simulink model "LQRC"  (R2020a)
settings: Solver=VariableStepAuto  StartTime=0  StopTime=30  FixedStep=0.01  MaxStep=0.1  MinStep=0.001  RelTol=1e-3  EnableMultiTasking=on
settings Model: Creator=s4khosra  LastModifiedBy=sashasen
settings DataIOCC: LimitDataPoints=on  SaveFormat=Array  ReturnWorkspaceOutputs=off
settings OptimizationCC: ExpressionDepthLimit=2147483647  LifeSpan=inf
settings DebuggingCC: AlgebraicLoopMsg=none  UnderspecifiedInitializationDetection=Classic  MergeDetectMultiDrivingBlocksExec=none  SolverPrmCheckMsg=warning  FcnCallInpInsideContextMsg=warning  AllowSymbolicDim=off  StateNameClashWarn=warning  SFUnexpectedBacktrackingDiag=warning  SFNoUnconditionalDefaultTransitionDiag=warning  SFExecutionAtInitializationDiag=none  ArithmeticOperatorsInVariantConditions=warning
settings HardwareCC: ProdBitPerPointer=32  ProdBitPerSizeT=32  ProdBitPerPtrDiffT=32  ProdLargestAtomicFloat=None  ProdIntDivRoundTo=Undefined  ProdEndianess=Unspecified  ProdWordSize=32  ProdHWDeviceType=32-bit Generic
settings ModelReferenceCC: PropagateSignalLabelsOutOfModel=off
settings SFSimCC: SimUseLocalCustomCode=off  CustomCodeUndefinedFunction=UseInterfaceOnly
settings RTWCC: RTWUseLocalCustomCode=off
settings CodeAppCC: StateflowObjectComments=on
settings GRTTargetCC: TargetLangStandard=C89/C90 (ANSI)  CombineOutputUpdateFcns=off  GRTInterface=on
settings ConfigComp: CovMetricSettings=dw  CovSaveCumulativeToWorkspaceVar=on  CovSaveSingleToWorkspaceVar=on  CovExternalEMLEnable=off  CovSFcnEnable=off

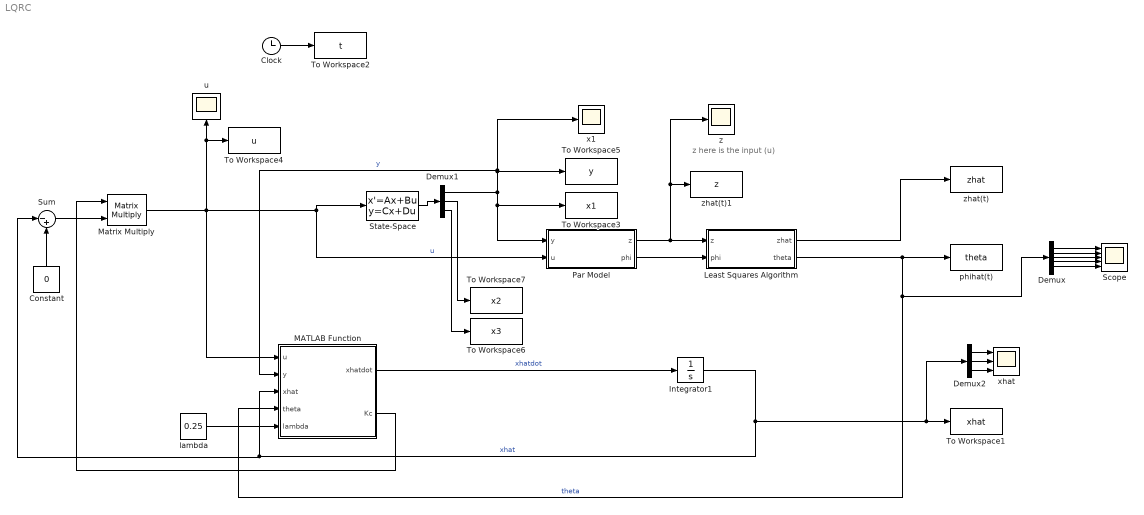
== system LQRC ==
  note: z here is the input (u)
  Clock : Clock
  Constant : Constant  Value=0
  Demux : Demux  Outputs=5
  Demux1 : Demux  Outputs=3
  Demux2 : Demux  Outputs=3
  Integrator1 : Integrator  InitialCondition=[1;-1;1]
  Least Squares Algorithm : Subsystem  TreatAsAtomicUnit=on
  MATLAB Function : MATLAB Function  TreatAsAtomicUnit=on
  Matrix Multiply : Product  Multiplication=Matrix(*)
  Par Model : Subsystem  TreatAsAtomicUnit=on
  Scope : Scope  NumInputPorts=5
  State-Space : StateSpace  A=[0.5 1 0 ;1 0 1; -0.5 0 0]  B=[2;2;1]  C=[1 0 0;0 1 0; 0 0 1]  D=[0;0;0]  InitialCondition=[1;-1;1]
  Sum : Sum  Inputs=|-+
  To Workspace1 : ToWorkspace  VariableName=xhat  SampleTime=-1
  To Workspace2 : ToWorkspace  VariableName=t  SampleTime=-1
  To Workspace3 : ToWorkspace  VariableName=x1  SampleTime=-1
  To Workspace4 : ToWorkspace  VariableName=u  SampleTime=-1
  To Workspace5 : ToWorkspace  VariableName=y  SampleTime=-1
  To Workspace6 : ToWorkspace  VariableName=x3  SampleTime=-1
  To Workspace7 : ToWorkspace  VariableName=x2  SampleTime=-1
  lambda : Constant  Value=0.25
  phihat(t) : ToWorkspace  VariableName=theta  SampleTime=-1
  u : Scope
  x1 : Scope
  xhat : Scope  NumInputPorts=3
  z : Scope
  zhat(t) : ToWorkspace  VariableName=zhat  SampleTime=-1
  zhat(t)1 : ToWorkspace  VariableName=z  SampleTime=-1
  wires:
  MATLAB Function/1(xhatdot) -> Integrator1/1  "xhatdot"
  Demux1/1 -> To Workspace3/1, Par Model/1(y), MATLAB Function/2(y), x1/1, To Workspace5/1  "y"
  Least Squares Algorithm/2(theta) -> MATLAB Function/4(theta), Demux/1, phihat(t)/1  "theta"
  Integrator1/1 -> Sum/1, MATLAB Function/3(xhat), Demux2/1, To Workspace1/1  "xhat"
  Clock/1 -> To Workspace2/1
  Par Model/1(z) -> zhat(t)1/1, z/1, Least Squares Algorithm/1(z)
  Least Squares Algorithm/1(zhat) -> zhat(t)/1
  Par Model/2(phi) -> Least Squares Algorithm/2(phi)
  Demux/1 -> Scope/1
  Demux/2 -> Scope/2
  Demux/3 -> Scope/3
  Demux/4 -> Scope/4
  Demux/5 -> Scope/5
  Matrix Multiply/1 -> MATLAB Function/1(u), u/1, To Workspace4/1, State-Space/1, Par Model/2(u)  "u"
  Demux2/1 -> xhat/1
  Demux2/2 -> xhat/2
  Demux2/3 -> xhat/3
  lambda/1 -> MATLAB Function/5(lambda)
  MATLAB Function/2(Kc) -> Matrix Multiply/1
  State-Space/1 -> Demux1/1
  Demux1/2 -> To Workspace7/1
  Demux1/3 -> To Workspace6/1
  Constant/1 -> Sum/2
  Sum/1 -> Matrix Multiply/2

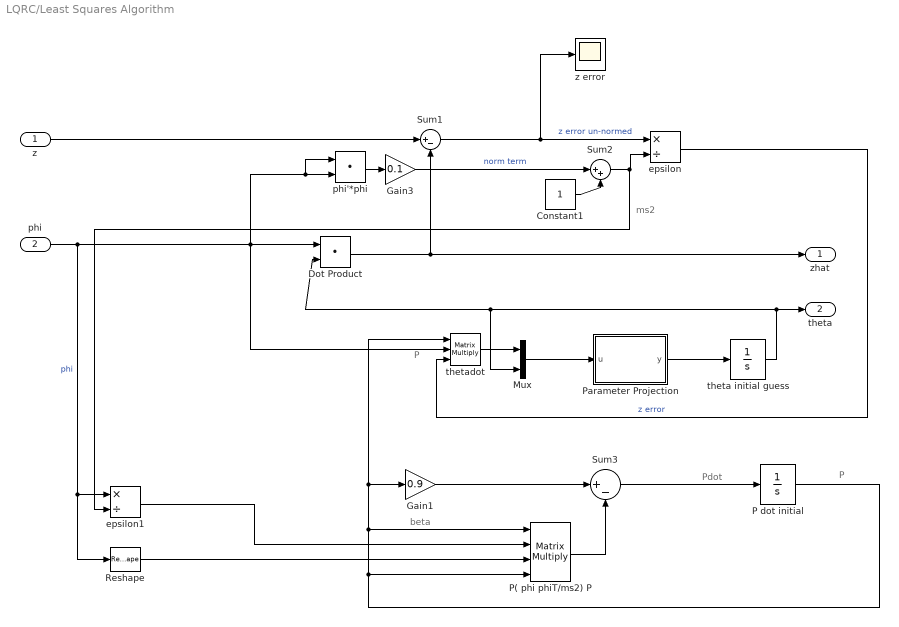
== system LQRC/Least Squares Algorithm ==
  note: P
  note: Pdot
  note: ms2
  note: beta
  note: P
  z : Inport
  phi : Inport  Port=2
  Constant1 : Constant
  Dot Product : DotProduct  InputSameDT=on  OutDataTypeStr=Inherit: Inherit via internal rule
  Gain1 : Gain  Gain=0.9
  Gain3 : Gain  Gain=0.1
  Mux : Mux  Inputs=2
  P dot initial : Integrator  InitialCondition=eye(5)
  P( phi phiT/ms2) P : Product  Inputs=4  Multiplication=Matrix(*)
  Parameter Projection : MATLAB Function  TreatAsAtomicUnit=on
  Reshape : Reshape  OutputDimensionality=Row vector (2-D)
  Sum1 : Sum  Inputs=|+-
  Sum2 : Sum  Inputs=|++
  Sum3 : Sum  Inputs=|+-
  epsilon : Product  Inputs=*/
  epsilon1 : Product  Inputs=*/
  phi'*phi : DotProduct  InputSameDT=on  OutDataTypeStr=Inherit: Inherit via internal rule
  theta initial guess : Integrator  InitialCondition=[0.01 0.01 0.01 0.01 0.01]
  thetadot : Product  Inputs=3  Multiplication=Matrix(*)
  z error : Scope
  zhat : Outport
  theta : Outport  Port=2
  wires:
  phi/1 -> Reshape/1, epsilon1/1, thetadot/2, phi'*phi/1, phi'*phi/2, Dot Product/1  "phi"
  z/1 -> Sum1/1
  Dot Product/1 -> zhat/1, Sum1/2
  theta initial guess/1 -> theta/1, Mux/2, Dot Product/2
  P dot initial/1 -> thetadot/1, Gain1/1, P( phi phiT/ms2) P/1, P( phi phiT/ms2) P/4
  phi'*phi/1 -> Gain3/1
  Gain3/1 -> Sum2/1  "norm term"
  Constant1/1 -> Sum2/2
  Sum2/1 -> epsilon1/2, epsilon/2
  Sum1/1 -> z error/1, epsilon/1  "z error un-normed"
  epsilon/1 -> thetadot/3  "z error"
  Gain1/1 -> Sum3/1
  Reshape/1 -> P( phi phiT/ms2) P/3
  epsilon1/1 -> P( phi phiT/ms2) P/2
  P( phi phiT/ms2) P/1 -> Sum3/2
  Sum3/1 -> P dot initial/1
  Parameter Projection/1(y) -> theta initial guess/1
  thetadot/1 -> Mux/1
  Mux/1 -> Parameter Projection/1(u)

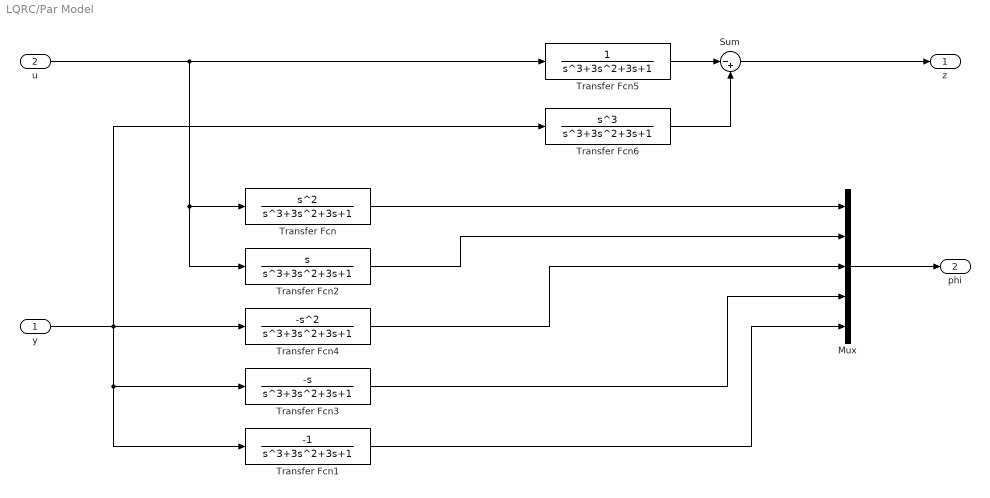
== system LQRC/Par Model ==
  y : Inport
  u : Inport  Port=2
  Mux : Mux  Inputs=5
  Sum : Sum  Inputs=|-+
  Transfer Fcn : TransferFcn  Numerator=[1 0 0]  Denominator=[1 3 3 1]
  Transfer Fcn1 : TransferFcn  Numerator=[-1]  Denominator=[1 3 3 1]
  Transfer Fcn2 : TransferFcn  Numerator=[1 0]  Denominator=[1 3 3 1]
  Transfer Fcn3 : TransferFcn  Numerator=[-1 0]  Denominator=[1 3 3 1]
  Transfer Fcn4 : TransferFcn  Numerator=[-1 0 0]  Denominator=[1 3 3 1]
  Transfer Fcn5 : TransferFcn  Denominator=[1 3 3 1]
  Transfer Fcn6 : TransferFcn  Numerator=[1 0 0 0]  Denominator=[1 3 3 1]
  z : Outport
  phi : Outport  Port=2
  wires:
  u/1 -> Transfer Fcn2/1, Transfer Fcn/1, Transfer Fcn5/1
  y/1 -> Transfer Fcn1/1, Transfer Fcn3/1, Transfer Fcn6/1, Transfer Fcn4/1
  Transfer Fcn5/1 -> Sum/1
  Transfer Fcn6/1 -> Sum/2
  Sum/1 -> z/1
  Mux/1 -> phi/1
  Transfer Fcn/1 -> Mux/1
  Transfer Fcn3/1 -> Mux/4
  Transfer Fcn1/1 -> Mux/5
  Transfer Fcn4/1 -> Mux/3
  Transfer Fcn2/1 -> Mux/2

== matlab function LQRC/Least Squares Algorithm/Parameter Projection ==
  data: u input; y output
function y = fcn(u)
%#codegen
n=5;
% lower bound b2 and b1 with 0
lb=[0 0 -1000 -1000 -1000];
ub=[1000 1000 1000 1000 1000];
u=u(:);
thetadot=u(1:n);
theta=u((n+1):(2*n));
y = thetadot;
for k=1:n,
    if (theta(k)<=lb(k)) & (thetadot(k)<0),
        y(k)=0;
    elseif (theta(k)>=ub(k)) & (thetadot(k)>0),
        y(k)=0;
    end
end

== matlab function LQRC/MATLAB Function ==
  data: u input; xhatdot output; y input; xhat input; theta input; lambda input; Kc output
function [xhatdot, Kc] = fcn(u,y,xhat,theta,lambda)

b2=theta(1);
b1=theta(2);
a2=theta(3);
a1=theta(4);
a0=theta(5);

Ko=[12-a2;48-a1;64-a0];
A=[-a2 1 0; -a1 0 1; -a0 0 0];
B=[b2; b1; 1];
% have xhat(1) here because C = [1 0 0]
xhatdot=A*xhat+B*u+Ko*(y-xhat(1));

coder.extrinsic('icare');
C = [1 0 0];
P = zeros(3,3);
Q = C*C';
Kc = [1 1 1];

[P,~,~] = icare(A, B, Q, lambda, zeros(3,1), eye(3), zeros(3,3));
Kc = (inv(lambda)*B)'*P;
